simulink model "model_observer_determine"  (R2024a)
settings: Solver=FixedStepAuto  StartTime=0.0  StopTime=10.0  FixedStep=0.0001  RelTol=1e-3
undefined symbols (not defined in the file): A, C, L, white_noise_var, x0, x_hat0
settings Model: Creator=anton  LastModifiedBy=anton

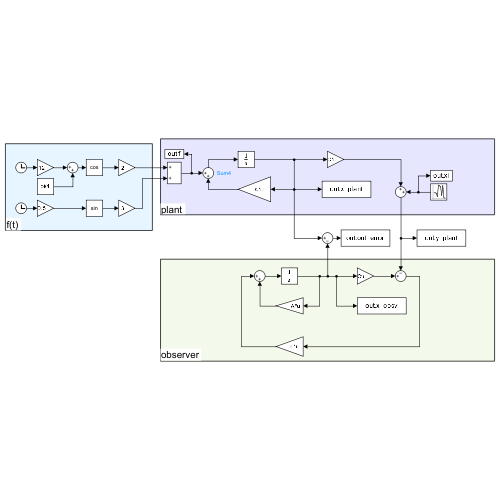
[thumbnail: Simulink's stored preview of the top-level diagram]
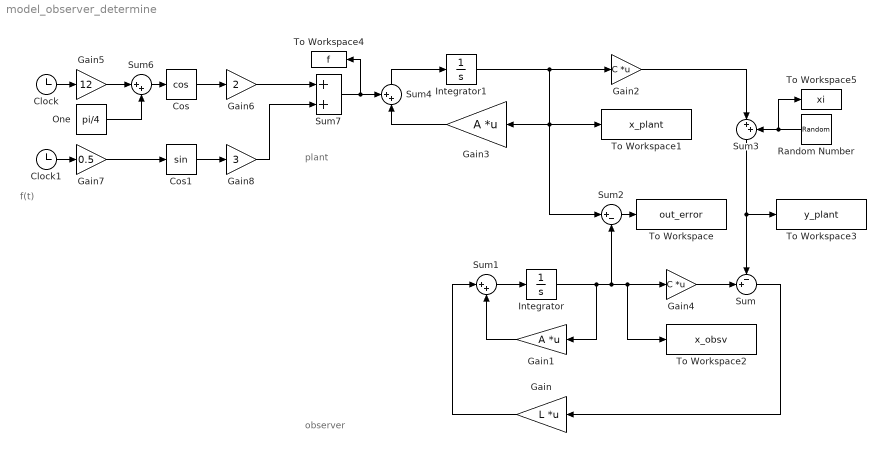
== system model_observer_determine ==
  note: f(t)
  note: observer
  note: plant
  Clock : Clock
  Clock1 : Clock
  Cos : Trigonometry  Operator=cos
  Cos1 : Trigonometry
  Gain : Gain  Gain=L  Multiplication=Matrix(K*u)
  Gain1 : Gain  Gain=A  Multiplication=Matrix(K*u)
  Gain2 : Gain  Gain=C  Multiplication=Matrix(K*u)
  Gain3 : Gain  Gain=A  Multiplication=Matrix(K*u)
  Gain4 : Gain  Gain=C  Multiplication=Matrix(K*u)
  Gain5 : Gain  Gain=12
  Gain6 : Gain  Gain=2
  Gain7 : Gain  Gain=0.5
  Gain8 : Gain  Gain=3
  Integrator : Integrator  InitialCondition=x_hat0
  Integrator1 : Integrator  InitialCondition=x0
  One : Constant  Value=pi/4  OutDataTypeStr=Inherit: Inherit via back propagation
  Random Number : RandomNumber  Variance=white_noise_var  SampleTime=0.0001
  Sum : Sum  Inputs=-+|
  Sum1 : Sum  Inputs=|++
  Sum2 : Sum  Inputs=|+-
  Sum3 : Sum  Inputs=|++
  Sum4 : Sum  Inputs=++|
  Sum6 : Sum  Inputs=|++
  Sum7 : Sum
  To Workspace : ToWorkspace  VariableName=out_error  SaveFormat=Timeseries  SampleTime=-1
  To Workspace1 : ToWorkspace  VariableName=x_plant  SaveFormat=Timeseries  SampleTime=-1
  To Workspace2 : ToWorkspace  VariableName=x_obsv  SaveFormat=Timeseries  SampleTime=-1
  To Workspace3 : ToWorkspace  VariableName=y_plant  SaveFormat=Timeseries  SampleTime=-1
  To Workspace4 : ToWorkspace  VariableName=f  SaveFormat=Timeseries  SampleTime=-1
  To Workspace5 : ToWorkspace  VariableName=xi  SaveFormat=Timeseries  SampleTime=-1
  wires:
  Sum/1 -> Gain/1
  Gain/1 -> Sum1/1
  Gain1/1 -> Sum1/2
  Sum1/1 -> Integrator/1
  Integrator/1 -> Gain1/1, Sum2/2, To Workspace2/1, Gain4/1
  Integrator1/1 -> Sum2/1, To Workspace1/1, Gain3/1, Gain2/1
  Gain4/1 -> Sum/2
  Sum2/1 -> To Workspace/1
  Gain2/1 -> Sum3/1
  Sum3/1 -> To Workspace3/1, Sum/1
  Random Number/1 -> To Workspace5/1, Sum3/2
  Gain3/1 -> Sum4/2
  Sum4/1 -> Integrator1/1
  Cos/1 -> Gain6/1
  Clock/1 -> Gain5/1
  Gain5/1 -> Sum6/1
  Sum6/1 -> Cos/1
  One/1 -> Sum6/2
  Cos1/1 -> Gain8/1
  Clock1/1 -> Gain7/1
  Gain7/1 -> Cos1/1
  Sum7/1 -> To Workspace4/1, Sum4/1
  Gain6/1 -> Sum7/1
  Gain8/1 -> Sum7/2
